simulink model "Asservissement_modele_simplifie"  (R2019b)
settings: Solver=VariableStepAuto  StartTime=0.0  StopTime=10.0  RelTol=1e-3
undefined symbols (not defined in the file): Cr, f, J, Km, R
libraries: simulink x1
settings Model: Creator=Shanly  LastModifiedBy=Shanly

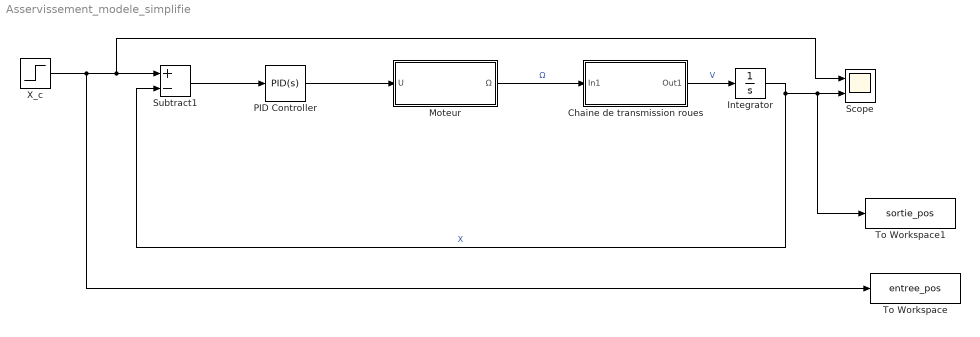
== system Asservissement_modele_simplifie ==
  Chaine de transmission roues : Subsystem
  Integrator : Integrator
  "Moteur " : Subsystem
  PID Controller : simulink/Continuous/PID Controller  Controller=PID  Form=Parallel  TimeDomain=Continuous-time  SampleTime=-1  IntegratorMethod=Forward Euler  FilterMethod=Forward Euler  ControllerParametersSource=internal  P=0.118673308674235  I=0.0073078914914254  D=0.290197564265985  UseFilter=on  N=986.48780438064  TunerSelectOption=Transfer Function Based (PID Tuner App)  InitialConditionSource=internal  InitialConditionForIntegrator=0  InitialConditionForFilter=0  DifferentiatorICPrevScaledInput=0  ExternalReset=none  TrackingMode=off  Kt=1  LimitOutput=off  UpperSaturationLimit=inf  LowerSaturationLimit=-inf  LinearizeAsGain=on  AntiWindupMode=none  Kb=1  POutMin=[]  POutMax=[]  IOutMin=[]  IOutMax=[]  DOutMin=[]  DOutMax=[]  NOutMin=[]  NOutMax=[]  SumOutMin=[]  SumOutMax=[]  SaturationOutMin=[]  SaturationOutMax=[]  PParamMin=[]  PParamMax=[]  IParamMin=[]  IParamMax=[]  DParamMin=[]  DParamMax=[]  NParamMin=[]  NParamMax=[]  KbParamMin=[]  KbParamMax=[]  KtParamMin=[]  KtParamMax=[]  KbOutMin=[]  KbOutMax=[]  KtOutMin=[]  KtOutMax=[]  IntegratorOutMin=[]  IntegratorOutMax=[]  FilterOutMin=[]  FilterOutMax=[]  SumI1OutMin=[]  SumI1OutMax=[]  SumI2OutMin=[]  SumI2OutMax=[]  SumI3OutMin=[]  SumI3OutMax=[]  SumI4OutMin=[]  SumI4OutMax=[]  SumDOutMin=[]  SumDOutMax=[]  DifferentiatorOutMin=[]  DifferentiatorOutMax=[]  FilterDiffOutCoefMin=[]  FilterDiffOutCoefMax=[]  ReciprocalOutMin=[]  ReciprocalOutMax=[]  SumDenOutMin=[]  SumDenOutMax=[]  SumNumOutMin=[]  SumNumOutMax=[]  DivideOutMin=[]  DivideOutMax=[]  IntegratorContinuousStateAttributes=''  IntegratorStateMustResolveToSignalObject=off  IntegratorRTWStateStorageClass=Auto  FilterContinuousStateAttributes=''  FilterStateMustResolveToSignalObject=off  FilterRTWStateStorageClass=Auto  ParallelPVariant=InternalParameters  IdealPVariant=Disabled  IVariant=InternalParameters  DVariant=InternalParameters  IntegratorVariant=Continuous  SatVariant=Disabled  AWVariant=Passthrough  PCopyVariant=Disabled  TRVariant=Disabled  FdbkBlocksVariant=Forward  IdealPFdbkVariant=Disabled  SatFdbkVariant=Disabled  DerivativeFilterVariant=ContFilter  NVariant=InternalParameters  NCopyVariant=Disabled  FilterICVariant=InternalICsFilter  IntegratorICVariant=InternalICs  ExternalResetVariant=Disabled  TRSumVariant=Passthrough  SumFdbkVariant=Disabled  SumVariant=Sum_PID
  Scope : Scope  NumInputPorts=2
  Subtract1 : Sum  Inputs=+-
  To Workspace : ToWorkspace  VariableName=entree_pos  SaveFormat=Timeseries  SampleTime=-1
  To Workspace1 : ToWorkspace  VariableName=sortie_pos  SaveFormat=Timeseries  SampleTime=-1
  X_c : Step  SampleTime=0
  wires:
  "Moteur "/1(Ω) -> Chaine de transmission roues/1(In1)  "Ω"
  PID Controller/1 -> "Moteur "/1(U)
  Chaine de transmission roues/1(Out1) -> Integrator/1  "V"
  Integrator/1 -> Subtract1/2, To Workspace1/1, Scope/2  "X"
  X_c/1 -> To Workspace/1, Scope/1, Subtract1/1
  Subtract1/1 -> PID Controller/1

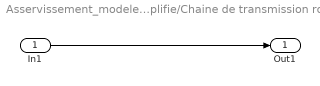
== system Asservissement_modele_simplifie/Chaine de transmission roues ==
  In1 : Inport
  Out1 : Outport
  wires:
  In1/1 -> Out1/1

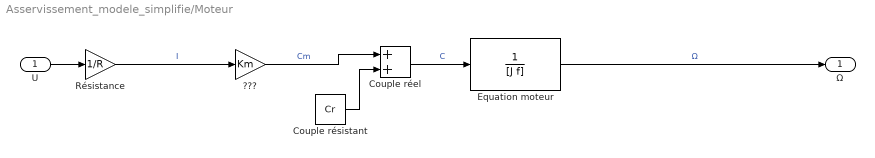
== system Asservissement_modele_simplifie/Moteur  ==
  U : Inport
  "???" : Gain  Gain=Km
  Couple réel : Sum
  Couple résistant : Constant  Value=Cr
  Equation moteur : TransferFcn  Denominator=[J f]
  Résistance : Gain  Gain=1/R
  Ω : Outport
  wires:
  U/1 -> Résistance/1
  Equation moteur/1 -> Ω/1  "Ω"
  Résistance/1 -> "???"/1  "I"
  "???"/1 -> Couple réel/1  "Cm"
  Couple réel/1 -> Equation moteur/1  "C"
  Couple résistant/1 -> Couple réel/2
